simulink model "filtros_r2015b"  (R2015b)
settings: Solver=VariableStepAuto  SolverMode=SingleTasking  StartTime=0.0  StopTime=10.0  RelTol=1e-3
libraries: dsparch4 x4
(part 3 of 5)

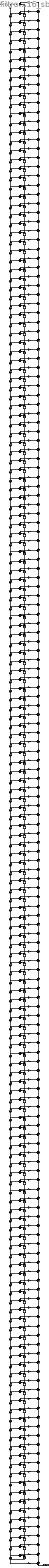
== system filtros_r2015b/filtro_bs_fir_direct_sym16_sb ==
  Input : Inport
  BodyDelayL{2..171} (170 alike) : Delay  DelayLength=1  InitialCondition=0
  BodyDelayR{2..171} (170 alike) : Delay  DelayLength=1  InitialCondition=0
  BodySumL{2..171} (170 alike) : Sum  Inputs=+|+  AccumDataTypeStr=fixdt(1,17,15)  OutDataTypeStr=fixdt(1,17,15)  RndMeth=Convergent
  BodySumR{2..171} (170 alike) : Sum  Inputs=++|  AccumDataTypeStr=fixdt(1,33,30)  OutDataTypeStr=fixdt(1,33,30)  RndMeth=Convergent
  ConvertIn : DataTypeConversion  OutDataTypeStr=fixdt(1,16,15)  RndMeth=Nearest  SaturateOnIntegerOverflow=on
  ConvertOut : DataTypeConversion  OutDataTypeStr=fixdt(1,33,30)  RndMeth=Convergent
  FootDelayL172 : Delay  DelayLength=1  InitialCondition=0
  FootSumR172 : Sum  Inputs=++|  AccumDataTypeStr=fixdt(1,33,30)  OutDataTypeStr=fixdt(1,33,30)  RndMeth=Convergent
  HeadDelayR1 : Delay  DelayLength=1  InitialCondition=0
  HeadSumL1 : Sum  Inputs=+|+  AccumDataTypeStr=fixdt(1,17,15)  OutDataTypeStr=fixdt(1,17,15)  RndMeth=Convergent
  h(1) : Gain  Gain=0.00222060902607300326  ParamDataTypeStr=fixdt(1,16,15)  OutDataTypeStr=fixdt(1,32,30)  RndMeth=Convergent
  h(10) : Gain  Gain=0.000412385856381775474  ParamDataTypeStr=fixdt(1,16,15)  OutDataTypeStr=fixdt(1,32,30)  RndMeth=Convergent
  h(100) : Gain  Gain=-0.00183683800817078082  ParamDataTypeStr=fixdt(1,16,15)  OutDataTypeStr=fixdt(1,32,30)  RndMeth=Convergent
  h(101) : Gain  Gain=-0.0108639596326587443  ParamDataTypeStr=fixdt(1,16,15)  OutDataTypeStr=fixdt(1,32,30)  RndMeth=Convergent
  h(102) : Gain  Gain=-0.00922719514825467643  ParamDataTypeStr=fixdt(1,16,15)  OutDataTypeStr=fixdt(1,32,30)  RndMeth=Convergent
  h(103) : Gain  Gain=0.00163747281524985618  ParamDataTypeStr=fixdt(1,16,15)  OutDataTypeStr=fixdt(1,32,30)  RndMeth=Convergent
  h(104) : Gain  Gain=0.0109887273848280828  ParamDataTypeStr=fixdt(1,16,15)  OutDataTypeStr=fixdt(1,32,30)  RndMeth=Convergent
  h(105) : Gain  Gain=0.00948674518474205107  ParamDataTypeStr=fixdt(1,16,15)  OutDataTypeStr=fixdt(1,32,30)  RndMeth=Convergent
  h(106) : Gain  Gain=-0.00138066436274078834  ParamDataTypeStr=fixdt(1,16,15)  OutDataTypeStr=fixdt(1,32,30)  RndMeth=Convergent
  h(107) : Gain  Gain=-0.0107847839373187305  ParamDataTypeStr=fixdt(1,16,15)  OutDataTypeStr=fixdt(1,32,30)  RndMeth=Convergent
  h(108) : Gain  Gain=-0.00943180866487196637  ParamDataTypeStr=fixdt(1,16,15)  OutDataTypeStr=fixdt(1,32,30)  RndMeth=Convergent
  h(109) : Gain  Gain=0.00112945650559354298  ParamDataTypeStr=fixdt(1,16,15)  OutDataTypeStr=fixdt(1,32,30)  RndMeth=Convergent
  h(11) : Gain  Gain=0.0012082136770825056  ParamDataTypeStr=fixdt(1,16,15)  OutDataTypeStr=fixdt(1,32,30)  RndMeth=Convergent
  h(110) : Gain  Gain=0.0102552016813565686  ParamDataTypeStr=fixdt(1,16,15)  OutDataTypeStr=fixdt(1,32,30)  RndMeth=Convergent
  h(111) : Gain  Gain=0.00900188398408828007  ParamDataTypeStr=fixdt(1,16,15)  OutDataTypeStr=fixdt(1,32,30)  RndMeth=Convergent
  h(112) : Gain  Gain=-0.000961145771569491512  ParamDataTypeStr=fixdt(1,16,15)  OutDataTypeStr=fixdt(1,32,30)  RndMeth=Convergent
  h(113) : Gain  Gain=-0.00942017850361522718  ParamDataTypeStr=fixdt(1,16,15)  OutDataTypeStr=fixdt(1,32,30)  RndMeth=Convergent
  h(114) : Gain  Gain=-0.00815339374212936327  ParamDataTypeStr=fixdt(1,16,15)  OutDataTypeStr=fixdt(1,32,30)  RndMeth=Convergent
  h(115) : Gain  Gain=0.00095452405654360248  ParamDataTypeStr=fixdt(1,16,15)  OutDataTypeStr=fixdt(1,32,30)  RndMeth=Convergent
  h(116) : Gain  Gain=0.00833604871664309077  ParamDataTypeStr=fixdt(1,16,15)  OutDataTypeStr=fixdt(1,32,30)  RndMeth=Convergent
  h(117) : Gain  Gain=0.00684396989036963662  ParamDataTypeStr=fixdt(1,16,15)  OutDataTypeStr=fixdt(1,32,30)  RndMeth=Convergent
  h(118) : Gain  Gain=-0.00119242778209114773  ParamDataTypeStr=fixdt(1,16,15)  OutDataTypeStr=fixdt(1,32,30)  RndMeth=Convergent
  h(119) : Gain  Gain=-0.00705305906451382351  ParamDataTypeStr=fixdt(1,16,15)  OutDataTypeStr=fixdt(1,32,30)  RndMeth=Convergent
  h(12) : Gain  Gain=0.000708848931376692445  ParamDataTypeStr=fixdt(1,16,15)  OutDataTypeStr=fixdt(1,32,30)  RndMeth=Convergent
  h(120) : Gain  Gain=-0.00507403810665585982  ParamDataTypeStr=fixdt(1,16,15)  OutDataTypeStr=fixdt(1,32,30)  RndMeth=Convergent
  h(121) : Gain  Gain=0.0017485040122219755  ParamDataTypeStr=fixdt(1,16,15)  OutDataTypeStr=fixdt(1,32,30)  RndMeth=Convergent
  h(122) : Gain  Gain=0.00566182762167975924  ParamDataTypeStr=fixdt(1,16,15)  OutDataTypeStr=fixdt(1,32,30)  RndMeth=Convergent
  h(123) : Gain  Gain=0.00285652374535125047  ParamDataTypeStr=fixdt(1,16,15)  OutDataTypeStr=fixdt(1,32,30)  RndMeth=Convergent
  h(124) : Gain  Gain=-0.00269106070621181808  ParamDataTypeStr=fixdt(1,16,15)  OutDataTypeStr=fixdt(1,32,30)  RndMeth=Convergent
  h(125) : Gain  Gain=-0.00424817527831348931  ParamDataTypeStr=fixdt(1,16,15)  OutDataTypeStr=fixdt(1,32,30)  RndMeth=Convergent
  h(126) : Gain  Gain=-0.000229684832746667594  ParamDataTypeStr=fixdt(1,16,15)  OutDataTypeStr=fixdt(1,32,30)  RndMeth=Convergent
  h(127) : Gain  Gain=0.00407093661353082233  ParamDataTypeStr=fixdt(1,16,15)  OutDataTypeStr=fixdt(1,32,30)  RndMeth=Convergent
  h(128) : Gain  Gain=0.00291483498180524067  ParamDataTypeStr=fixdt(1,16,15)  OutDataTypeStr=fixdt(1,32,30)  RndMeth=Convergent
  h(129) : Gain  Gain=-0.00274240933992378781  ParamDataTypeStr=fixdt(1,16,15)  OutDataTypeStr=fixdt(1,32,30)  RndMeth=Convergent
  h(13) : Gain  Gain=-0.000527267715872998242  ParamDataTypeStr=fixdt(1,16,15)  OutDataTypeStr=fixdt(1,32,30)  RndMeth=Convergent
  h(130) : Gain  Gain=-0.00591588442091149896  ParamDataTypeStr=fixdt(1,16,15)  OutDataTypeStr=fixdt(1,32,30)  RndMeth=Convergent
  h(131) : Gain  Gain=-0.0017616838703545161  ParamDataTypeStr=fixdt(1,16,15)  OutDataTypeStr=fixdt(1,32,30)  RndMeth=Convergent
  h(132) : Gain  Gain=0.00597490325309535299  ParamDataTypeStr=fixdt(1,16,15)  OutDataTypeStr=fixdt(1,32,30)  RndMeth=Convergent
  h(133) : Gain  Gain=0.00823416750476205564  ParamDataTypeStr=fixdt(1,16,15)  OutDataTypeStr=fixdt(1,32,30)  RndMeth=Convergent
  h(134) : Gain  Gain=0.000885427072030269056  ParamDataTypeStr=fixdt(1,16,15)  OutDataTypeStr=fixdt(1,32,30)  RndMeth=Convergent
  h(135) : Gain  Gain=-0.0093650338513660801  ParamDataTypeStr=fixdt(1,16,15)  OutDataTypeStr=fixdt(1,32,30)  RndMeth=Convergent
  h(136) : Gain  Gain=-0.0110087803321226481  ParamDataTypeStr=fixdt(1,16,15)  OutDataTypeStr=fixdt(1,32,30)  RndMeth=Convergent
  h(137) : Gain  Gain=-0.000374405366293637204  ParamDataTypeStr=fixdt(1,16,15)  OutDataTypeStr=fixdt(1,32,30)  RndMeth=Convergent
  h(138) : Gain  Gain=0.0127923118217058915  ParamDataTypeStr=fixdt(1,16,15)  OutDataTypeStr=fixdt(1,32,30)  RndMeth=Convergent
  h(139) : Gain  Gain=0.0141925500900669105  ParamDataTypeStr=fixdt(1,16,15)  OutDataTypeStr=fixdt(1,32,30)  RndMeth=Convergent
  h(14) : Gain  Gain=-0.00115435994390551471  ParamDataTypeStr=fixdt(1,16,15)  OutDataTypeStr=fixdt(1,32,30)  RndMeth=Convergent
  h(140) : Gain  Gain=0.000297609131461152134  ParamDataTypeStr=fixdt(1,16,15)  OutDataTypeStr=fixdt(1,32,30)  RndMeth=Convergent
  h(141) : Gain  Gain=-0.0161298900491302633  ParamDataTypeStr=fixdt(1,16,15)  OutDataTypeStr=fixdt(1,32,30)  RndMeth=Convergent
  h(142) : Gain  Gain=-0.0177117572182131991  ParamDataTypeStr=fixdt(1,16,15)  OutDataTypeStr=fixdt(1,32,30)  RndMeth=Convergent
  h(143) : Gain  Gain=-0.00070122210733707406  ParamDataTypeStr=fixdt(1,16,15)  OutDataTypeStr=fixdt(1,32,30)  RndMeth=Convergent
  h(144) : Gain  Gain=0.0192516530564409392  ParamDataTypeStr=fixdt(1,16,15)  OutDataTypeStr=fixdt(1,32,30)  RndMeth=Convergent
  h(145) : Gain  Gain=0.0214725815198791338  ParamDataTypeStr=fixdt(1,16,15)  OutDataTypeStr=fixdt(1,32,30)  RndMeth=Convergent
  h(146) : Gain  Gain=0.00160886427991767172  ParamDataTypeStr=fixdt(1,16,15)  OutDataTypeStr=fixdt(1,32,30)  RndMeth=Convergent
  h(147) : Gain  Gain=-0.0220352330154781964  ParamDataTypeStr=fixdt(1,16,15)  OutDataTypeStr=fixdt(1,32,30)  RndMeth=Convergent
  h(148) : Gain  Gain=-0.0253625767260405761  ParamDataTypeStr=fixdt(1,16,15)  OutDataTypeStr=fixdt(1,32,30)  RndMeth=Convergent
  h(149) : Gain  Gain=-0.00302084071867347913  ParamDataTypeStr=fixdt(1,16,15)  OutDataTypeStr=fixdt(1,32,30)  RndMeth=Convergent
  h(15) : Gain  Gain=-0.000500072760209519418  ParamDataTypeStr=fixdt(1,16,15)  OutDataTypeStr=fixdt(1,32,30)  RndMeth=Convergent
  h(150) : Gain  Gain=0.0243632351958552353  ParamDataTypeStr=fixdt(1,16,15)  OutDataTypeStr=fixdt(1,32,30)  RndMeth=Convergent
  h(151) : Gain  Gain=0.0292458735180988298  ParamDataTypeStr=fixdt(1,16,15)  OutDataTypeStr=fixdt(1,32,30)  RndMeth=Convergent
  h(152) : Gain  Gain=0.00489806445322205682  ParamDataTypeStr=fixdt(1,16,15)  OutDataTypeStr=fixdt(1,32,30)  RndMeth=Convergent
  h(153) : Gain  Gain=-0.0261477012653955863  ParamDataTypeStr=fixdt(1,16,15)  OutDataTypeStr=fixdt(1,32,30)  RndMeth=Convergent
  h(154) : Gain  Gain=-0.0329897200285691264  ParamDataTypeStr=fixdt(1,16,15)  OutDataTypeStr=fixdt(1,32,30)  RndMeth=Convergent
  h(155) : Gain  Gain=-0.00718491130158882118  ParamDataTypeStr=fixdt(1,16,15)  OutDataTypeStr=fixdt(1,32,30)  RndMeth=Convergent
  h(156) : Gain  Gain=0.0273141193534726101  ParamDataTypeStr=fixdt(1,16,15)  OutDataTypeStr=fixdt(1,32,30)  RndMeth=Convergent
  h(157) : Gain  Gain=0.0364508104956247289  ParamDataTypeStr=fixdt(1,16,15)  OutDataTypeStr=fixdt(1,32,30)  RndMeth=Convergent
  h(158) : Gain  Gain=0.00979190705266517157  ParamDataTypeStr=fixdt(1,16,15)  OutDataTypeStr=fixdt(1,32,30)  RndMeth=Convergent
  h(159) : Gain  Gain=-0.0278216938080646271  ParamDataTypeStr=fixdt(1,16,15)  OutDataTypeStr=fixdt(1,32,30)  RndMeth=Convergent
  h(16) : Gain  Gain=0.000688761844683712598  ParamDataTypeStr=fixdt(1,16,15)  OutDataTypeStr=fixdt(1,32,30)  RndMeth=Convergent
  h(160) : Gain  Gain=-0.0394970137823456025  ParamDataTypeStr=fixdt(1,16,15)  OutDataTypeStr=fixdt(1,32,30)  RndMeth=Convergent
  h(161) : Gain  Gain=-0.0126125709016341354  ParamDataTypeStr=fixdt(1,16,15)  OutDataTypeStr=fixdt(1,32,30)  RndMeth=Convergent
  h(162) : Gain  Gain=0.0276570288609940609  ParamDataTypeStr=fixdt(1,16,15)  OutDataTypeStr=fixdt(1,32,30)  RndMeth=Convergent
  h(163) : Gain  Gain=0.0420062041083570439  ParamDataTypeStr=fixdt(1,16,15)  OutDataTypeStr=fixdt(1,32,30)  RndMeth=Convergent
  h(164) : Gain  Gain=0.0155224470683002526  ParamDataTypeStr=fixdt(1,16,15)  OutDataTypeStr=fixdt(1,32,30)  RndMeth=Convergent
  h(165) : Gain  Gain=-0.0268379125320710073  ParamDataTypeStr=fixdt(1,16,15)  OutDataTypeStr=fixdt(1,32,30)  RndMeth=Convergent
  h(166) : Gain  Gain=-0.0438767987017301478  ParamDataTypeStr=fixdt(1,16,15)  OutDataTypeStr=fixdt(1,32,30)  RndMeth=Convergent
  h(167) : Gain  Gain=-0.0183901617907575449  ParamDataTypeStr=fixdt(1,16,15)  OutDataTypeStr=fixdt(1,32,30)  RndMeth=Convergent
  h(168) : Gain  Gain=0.0254141122423833764  ParamDataTypeStr=fixdt(1,16,15)  OutDataTypeStr=fixdt(1,32,30)  RndMeth=Convergent
  h(169) : Gain  Gain=0.0450290877668963474  ParamDataTypeStr=fixdt(1,16,15)  OutDataTypeStr=fixdt(1,32,30)  RndMeth=Convergent
  h(17) : Gain  Gain=0.00107522738688104608  ParamDataTypeStr=fixdt(1,16,15)  OutDataTypeStr=fixdt(1,32,30)  RndMeth=Convergent
  h(170) : Gain  Gain=0.021081893690384497  ParamDataTypeStr=fixdt(1,16,15)  OutDataTypeStr=fixdt(1,32,30)  RndMeth=Convergent
  h(171) : Gain  Gain=-0.0234612272015558634  ParamDataTypeStr=fixdt(1,16,15)  OutDataTypeStr=fixdt(1,32,30)  RndMeth=Convergent
  h(172) : Gain  Gain=0.92844636087036847  ParamDataTypeStr=fixdt(1,16,15)  OutDataTypeStr=fixdt(1,32,30)  RndMeth=Convergent
  h(18) : Gain  Gain=0.00021708622303679784  ParamDataTypeStr=fixdt(1,16,15)  OutDataTypeStr=fixdt(1,32,30)  RndMeth=Convergent
  h(19) : Gain  Gain=-0.000907506893595811152  ParamDataTypeStr=fixdt(1,16,15)  OutDataTypeStr=fixdt(1,32,30)  RndMeth=Convergent
  h(2) : Gain  Gain=-0.0126542523812769661  ParamDataTypeStr=fixdt(1,16,15)  OutDataTypeStr=fixdt(1,32,30)  RndMeth=Convergent
  h(20) : Gain  Gain=-0.00098456841772494026  ParamDataTypeStr=fixdt(1,16,15)  OutDataTypeStr=fixdt(1,32,30)  RndMeth=Convergent
  h(21) : Gain  Gain=0.000135034611801735488  ParamDataTypeStr=fixdt(1,16,15)  OutDataTypeStr=fixdt(1,32,30)  RndMeth=Convergent
  h(22) : Gain  Gain=0.0011904117302944002  ParamDataTypeStr=fixdt(1,16,15)  OutDataTypeStr=fixdt(1,32,30)  RndMeth=Convergent
  h(23) : Gain  Gain=0.000897348105847610368  ParamDataTypeStr=fixdt(1,16,15)  OutDataTypeStr=fixdt(1,32,30)  RndMeth=Convergent
  h(24) : Gain  Gain=-0.000544809004851308965  ParamDataTypeStr=fixdt(1,16,15)  OutDataTypeStr=fixdt(1,32,30)  RndMeth=Convergent
  h(25) : Gain  Gain=-0.00153935391414636888  ParamDataTypeStr=fixdt(1,16,15)  OutDataTypeStr=fixdt(1,32,30)  RndMeth=Convergent
  h(26) : Gain  Gain=-0.000828005173735774504  ParamDataTypeStr=fixdt(1,16,15)  OutDataTypeStr=fixdt(1,32,30)  RndMeth=Convergent
  h(27) : Gain  Gain=0.000996889815879576074  ParamDataTypeStr=fixdt(1,16,15)  OutDataTypeStr=fixdt(1,32,30)  RndMeth=Convergent
  h(28) : Gain  Gain=0.0019514135346378515  ParamDataTypeStr=fixdt(1,16,15)  OutDataTypeStr=fixdt(1,32,30)  RndMeth=Convergent
  h(29) : Gain  Gain=0.000790406883380305979  ParamDataTypeStr=fixdt(1,16,15)  OutDataTypeStr=fixdt(1,32,30)  RndMeth=Convergent
  h(3) : Gain  Gain=-0.00285785975806639734  ParamDataTypeStr=fixdt(1,16,15)  OutDataTypeStr=fixdt(1,32,30)  RndMeth=Convergent
  h(30) : Gain  Gain=-0.00147057635761781201  ParamDataTypeStr=fixdt(1,16,15)  OutDataTypeStr=fixdt(1,32,30)  RndMeth=Convergent
  h(31) : Gain  Gain=-0.00241626228825247806  ParamDataTypeStr=fixdt(1,16,15)  OutDataTypeStr=fixdt(1,32,30)  RndMeth=Convergent
  h(32) : Gain  Gain=-0.00079322658642497451  ParamDataTypeStr=fixdt(1,16,15)  OutDataTypeStr=fixdt(1,32,30)  RndMeth=Convergent
  h(33) : Gain  Gain=0.00194526333770608968  ParamDataTypeStr=fixdt(1,16,15)  OutDataTypeStr=fixdt(1,32,30)  RndMeth=Convergent
  h(34) : Gain  Gain=0.0029194310934874913  ParamDataTypeStr=fixdt(1,16,15)  OutDataTypeStr=fixdt(1,32,30)  RndMeth=Convergent
  h(35) : Gain  Gain=0.000842470514714747172  ParamDataTypeStr=fixdt(1,16,15)  OutDataTypeStr=fixdt(1,32,30)  RndMeth=Convergent
  h(36) : Gain  Gain=-0.00239778430088512153  ParamDataTypeStr=fixdt(1,16,15)  OutDataTypeStr=fixdt(1,32,30)  RndMeth=Convergent
  h(37) : Gain  Gain=-0.00343927344050146957  ParamDataTypeStr=fixdt(1,16,15)  OutDataTypeStr=fixdt(1,32,30)  RndMeth=Convergent
  h(38) : Gain  Gain=-0.000936473940016707435  ParamDataTypeStr=fixdt(1,16,15)  OutDataTypeStr=fixdt(1,32,30)  RndMeth=Convergent
  h(39) : Gain  Gain=0.00280722916414461419  ParamDataTypeStr=fixdt(1,16,15)  OutDataTypeStr=fixdt(1,32,30)  RndMeth=Convergent
  h(4) : Gain  Gain=-6.27866860752195359e-05  ParamDataTypeStr=fixdt(1,16,15)  OutDataTypeStr=fixdt(1,32,30)  RndMeth=Convergent
  h(40) : Gain  Gain=0.00395010111825385129  ParamDataTypeStr=fixdt(1,16,15)  OutDataTypeStr=fixdt(1,32,30)  RndMeth=Convergent
  h(41) : Gain  Gain=0.00106808840411088692  ParamDataTypeStr=fixdt(1,16,15)  OutDataTypeStr=fixdt(1,32,30)  RndMeth=Convergent
  h(42) : Gain  Gain=-0.00315451566029618024  ParamDataTypeStr=fixdt(1,16,15)  OutDataTypeStr=fixdt(1,32,30)  RndMeth=Convergent
  h(43) : Gain  Gain=-0.00442195264195982887  ParamDataTypeStr=fixdt(1,16,15)  OutDataTypeStr=fixdt(1,32,30)  RndMeth=Convergent
  h(44) : Gain  Gain=-0.00122255919972922753  ParamDataTypeStr=fixdt(1,16,15)  OutDataTypeStr=fixdt(1,32,30)  RndMeth=Convergent
  h(45) : Gain  Gain=0.00342517772747777133  ParamDataTypeStr=fixdt(1,16,15)  OutDataTypeStr=fixdt(1,32,30)  RndMeth=Convergent
  h(46) : Gain  Gain=0.00482320302455260287  ParamDataTypeStr=fixdt(1,16,15)  OutDataTypeStr=fixdt(1,32,30)  RndMeth=Convergent
  h(47) : Gain  Gain=0.00137963206631302971  ParamDataTypeStr=fixdt(1,16,15)  OutDataTypeStr=fixdt(1,32,30)  RndMeth=Convergent
  h(48) : Gain  Gain=-0.00361108914948540588  ParamDataTypeStr=fixdt(1,16,15)  OutDataTypeStr=fixdt(1,32,30)  RndMeth=Convergent
  h(49) : Gain  Gain=-0.0051234196132662101  ParamDataTypeStr=fixdt(1,16,15)  OutDataTypeStr=fixdt(1,32,30)  RndMeth=Convergent
  h(5) : Gain  Gain=0.0011441808540458725  ParamDataTypeStr=fixdt(1,16,15)  OutDataTypeStr=fixdt(1,32,30)  RndMeth=Convergent
  h(50) : Gain  Gain=-0.00151391720299139305  ParamDataTypeStr=fixdt(1,16,15)  OutDataTypeStr=fixdt(1,32,30)  RndMeth=Convergent
  h(51) : Gain  Gain=0.00370986731030357791  ParamDataTypeStr=fixdt(1,16,15)  OutDataTypeStr=fixdt(1,32,30)  RndMeth=Convergent
  h(52) : Gain  Gain=0.00529509616594016613  ParamDataTypeStr=fixdt(1,16,15)  OutDataTypeStr=fixdt(1,32,30)  RndMeth=Convergent
  h(53) : Gain  Gain=0.00159648812698948606  ParamDataTypeStr=fixdt(1,16,15)  OutDataTypeStr=fixdt(1,32,30)  RndMeth=Convergent
  h(54) : Gain  Gain=-0.00373099483536572154  ParamDataTypeStr=fixdt(1,16,15)  OutDataTypeStr=fixdt(1,32,30)  RndMeth=Convergent
  h(55) : Gain  Gain=-0.00532117775878846073  ParamDataTypeStr=fixdt(1,16,15)  OutDataTypeStr=fixdt(1,32,30)  RndMeth=Convergent
  h(56) : Gain  Gain=-0.00159242660687583873  ParamDataTypeStr=fixdt(1,16,15)  OutDataTypeStr=fixdt(1,32,30)  RndMeth=Convergent
  h(57) : Gain  Gain=0.00367945523701494748  ParamDataTypeStr=fixdt(1,16,15)  OutDataTypeStr=fixdt(1,32,30)  RndMeth=Convergent
  h(58) : Gain  Gain=0.0052061653709269606  ParamDataTypeStr=fixdt(1,16,15)  OutDataTypeStr=fixdt(1,32,30)  RndMeth=Convergent
  h(59) : Gain  Gain=0.00147157392126652845  ParamDataTypeStr=fixdt(1,16,15)  OutDataTypeStr=fixdt(1,32,30)  RndMeth=Convergent
  h(6) : Gain  Gain=0.000896258283817716328  ParamDataTypeStr=fixdt(1,16,15)  OutDataTypeStr=fixdt(1,32,30)  RndMeth=Convergent
  h(60) : Gain  Gain=-0.00361588185118073922  ParamDataTypeStr=fixdt(1,16,15)  OutDataTypeStr=fixdt(1,32,30)  RndMeth=Convergent
  h(61) : Gain  Gain=-0.00490141555871920903  ParamDataTypeStr=fixdt(1,16,15)  OutDataTypeStr=fixdt(1,32,30)  RndMeth=Convergent
  h(62) : Gain  Gain=-0.00121047830165690374  ParamDataTypeStr=fixdt(1,16,15)  OutDataTypeStr=fixdt(1,32,30)  RndMeth=Convergent
  h(63) : Gain  Gain=0.00352542594050439051  ParamDataTypeStr=fixdt(1,16,15)  OutDataTypeStr=fixdt(1,32,30)  RndMeth=Convergent
  h(64) : Gain  Gain=0.00445284916134371014  ParamDataTypeStr=fixdt(1,16,15)  OutDataTypeStr=fixdt(1,32,30)  RndMeth=Convergent
  h(65) : Gain  Gain=0.000791426268911049158  ParamDataTypeStr=fixdt(1,16,15)  OutDataTypeStr=fixdt(1,32,30)  RndMeth=Convergent
  h(66) : Gain  Gain=-0.00345955811828613236  ParamDataTypeStr=fixdt(1,16,15)  OutDataTypeStr=fixdt(1,32,30)  RndMeth=Convergent
  h(67) : Gain  Gain=-0.00386295620000698219  ParamDataTypeStr=fixdt(1,16,15)  OutDataTypeStr=fixdt(1,32,30)  RndMeth=Convergent
  h(68) : Gain  Gain=-0.000195973685172349036  ParamDataTypeStr=fixdt(1,16,15)  OutDataTypeStr=fixdt(1,32,30)  RndMeth=Convergent
  h(69) : Gain  Gain=0.00344274784340699606  ParamDataTypeStr=fixdt(1,16,15)  OutDataTypeStr=fixdt(1,32,30)  RndMeth=Convergent
  h(7) : Gain  Gain=-0.000331426495396970144  ParamDataTypeStr=fixdt(1,16,15)  OutDataTypeStr=fixdt(1,32,30)  RndMeth=Convergent
  h(70) : Gain  Gain=0.00315382863405564307  ParamDataTypeStr=fixdt(1,16,15)  OutDataTypeStr=fixdt(1,32,30)  RndMeth=Convergent
  h(71) : Gain  Gain=-0.000582376133074710006  ParamDataTypeStr=fixdt(1,16,15)  OutDataTypeStr=fixdt(1,32,30)  RndMeth=Convergent
  h(72) : Gain  Gain=-0.00351181599169146652  ParamDataTypeStr=fixdt(1,16,15)  OutDataTypeStr=fixdt(1,32,30)  RndMeth=Convergent
  h(73) : Gain  Gain=-0.00236215784465629297  ParamDataTypeStr=fixdt(1,16,15)  OutDataTypeStr=fixdt(1,32,30)  RndMeth=Convergent
  h(74) : Gain  Gain=0.00153579939763267333  ParamDataTypeStr=fixdt(1,16,15)  OutDataTypeStr=fixdt(1,32,30)  RndMeth=Convergent
  h(75) : Gain  Gain=0.00370136458943965373  ParamDataTypeStr=fixdt(1,16,15)  OutDataTypeStr=fixdt(1,32,30)  RndMeth=Convergent
  h(76) : Gain  Gain=0.00154425151614053543  ParamDataTypeStr=fixdt(1,16,15)  OutDataTypeStr=fixdt(1,32,30)  RndMeth=Convergent
  h(77) : Gain  Gain=-0.00262336900807332929  ParamDataTypeStr=fixdt(1,16,15)  OutDataTypeStr=fixdt(1,32,30)  RndMeth=Convergent
  h(78) : Gain  Gain=-0.00400604629593016501  ParamDataTypeStr=fixdt(1,16,15)  OutDataTypeStr=fixdt(1,32,30)  RndMeth=Convergent
  h(79) : Gain  Gain=-0.000720258293274521409  ParamDataTypeStr=fixdt(1,16,15)  OutDataTypeStr=fixdt(1,32,30)  RndMeth=Convergent
  h(8) : Gain  Gain=-0.00122625529434006045  ParamDataTypeStr=fixdt(1,16,15)  OutDataTypeStr=fixdt(1,32,30)  RndMeth=Convergent
  h(80) : Gain  Gain=0.00383463380064707733  ParamDataTypeStr=fixdt(1,16,15)  OutDataTypeStr=fixdt(1,32,30)  RndMeth=Convergent
  h(81) : Gain  Gain=0.00445475536974668761  ParamDataTypeStr=fixdt(1,16,15)  OutDataTypeStr=fixdt(1,32,30)  RndMeth=Convergent
  h(82) : Gain  Gain=-4.60177465353575697e-05  ParamDataTypeStr=fixdt(1,16,15)  OutDataTypeStr=fixdt(1,32,30)  RndMeth=Convergent
  h(83) : Gain  Gain=-0.00510941162252769206  ParamDataTypeStr=fixdt(1,16,15)  OutDataTypeStr=fixdt(1,32,30)  RndMeth=Convergent
  h(84) : Gain  Gain=-0.00503113887403160848  ParamDataTypeStr=fixdt(1,16,15)  OutDataTypeStr=fixdt(1,32,30)  RndMeth=Convergent
  h(85) : Gain  Gain=0.000719907321048572049  ParamDataTypeStr=fixdt(1,16,15)  OutDataTypeStr=fixdt(1,32,30)  RndMeth=Convergent
  h(86) : Gain  Gain=0.00639742929747593846  ParamDataTypeStr=fixdt(1,16,15)  OutDataTypeStr=fixdt(1,32,30)  RndMeth=Convergent
  h(87) : Gain  Gain=0.00571934912806121212  ParamDataTypeStr=fixdt(1,16,15)  OutDataTypeStr=fixdt(1,32,30)  RndMeth=Convergent
  h(88) : Gain  Gain=-0.00126357426321187542  ParamDataTypeStr=fixdt(1,16,15)  OutDataTypeStr=fixdt(1,32,30)  RndMeth=Convergent
  h(89) : Gain  Gain=-0.00763605641798632221  ParamDataTypeStr=fixdt(1,16,15)  OutDataTypeStr=fixdt(1,32,30)  RndMeth=Convergent
  h(9) : Gain  Gain=-0.000842143561281415501  ParamDataTypeStr=fixdt(1,16,15)  OutDataTypeStr=fixdt(1,32,30)  RndMeth=Convergent
  h(90) : Gain  Gain=-0.00648525362000833966  ParamDataTypeStr=fixdt(1,16,15)  OutDataTypeStr=fixdt(1,32,30)  RndMeth=Convergent
  h(91) : Gain  Gain=0.00165155190893082971  ParamDataTypeStr=fixdt(1,16,15)  OutDataTypeStr=fixdt(1,32,30)  RndMeth=Convergent
  h(92) : Gain  Gain=0.00876118917065600751  ParamDataTypeStr=fixdt(1,16,15)  OutDataTypeStr=fixdt(1,32,30)  RndMeth=Convergent
  h(93) : Gain  Gain=0.0072820300968526562  ParamDataTypeStr=fixdt(1,16,15)  OutDataTypeStr=fixdt(1,32,30)  RndMeth=Convergent
  h(94) : Gain  Gain=-0.00187150944773054636  ParamDataTypeStr=fixdt(1,16,15)  OutDataTypeStr=fixdt(1,32,30)  RndMeth=Convergent
  h(95) : Gain  Gain=-0.00971025998510001952  ParamDataTypeStr=fixdt(1,16,15)  OutDataTypeStr=fixdt(1,32,30)  RndMeth=Convergent
  h(96) : Gain  Gain=-0.00805071853330361492  ParamDataTypeStr=fixdt(1,16,15)  OutDataTypeStr=fixdt(1,32,30)  RndMeth=Convergent
  h(97) : Gain  Gain=0.00192657035016093937  ParamDataTypeStr=fixdt(1,16,15)  OutDataTypeStr=fixdt(1,32,30)  RndMeth=Convergent
  h(98) : Gain  Gain=0.0104266340022652303  ParamDataTypeStr=fixdt(1,16,15)  OutDataTypeStr=fixdt(1,32,30)  RndMeth=Convergent
  h(99) : Gain  Gain=0.00872346674455828572  ParamDataTypeStr=fixdt(1,16,15)  OutDataTypeStr=fixdt(1,32,30)  RndMeth=Convergent
  Output : Outport
  wires:
  Input/1 -> ConvertIn/1
  HeadSumL1/1 -> h(1)/1
  h(1)/1 -> BodySumR2/2
  HeadDelayR1/1 -> HeadSumL1/2
  ConvertIn/1 -> HeadSumL1/1, BodyDelayL2/1
  BodyDelayL2/1 -> BodySumL2/1, BodyDelayL3/1
  BodySumL2/1 -> h(2)/1
  h(2)/1 -> BodySumR2/1
  BodyDelayR2/1 -> BodySumL2/2, HeadDelayR1/1
  BodySumR2/1 -> BodySumR3/2
  BodyDelayL3/1 -> BodySumL3/1, BodyDelayL4/1
  BodySumL3/1 -> h(3)/1
  h(3)/1 -> BodySumR3/1
  BodyDelayR3/1 -> BodySumL3/2, BodyDelayR2/1
  BodySumR3/1 -> BodySumR4/2
  BodyDelayL4/1 -> BodySumL4/1, BodyDelayL5/1
  BodySumL4/1 -> h(4)/1
  h(4)/1 -> BodySumR4/1
  BodyDelayR4/1 -> BodySumL4/2, BodyDelayR3/1
  BodySumR4/1 -> BodySumR5/2
  BodyDelayL5/1 -> BodySumL5/1, BodyDelayL6/1
  BodySumL5/1 -> h(5)/1
  h(5)/1 -> BodySumR5/1
  BodyDelayR5/1 -> BodySumL5/2, BodyDelayR4/1
  BodySumR5/1 -> BodySumR6/2
  BodyDelayL6/1 -> BodySumL6/1, BodyDelayL7/1
  BodySumL6/1 -> h(6)/1
  h(6)/1 -> BodySumR6/1
  BodyDelayR6/1 -> BodySumL6/2, BodyDelayR5/1
  BodySumR6/1 -> BodySumR7/2
  BodyDelayL7/1 -> BodySumL7/1, BodyDelayL8/1
  BodySumL7/1 -> h(7)/1
  h(7)/1 -> BodySumR7/1
  BodyDelayR7/1 -> BodySumL7/2, BodyDelayR6/1
  BodySumR7/1 -> BodySumR8/2
  BodyDelayL8/1 -> BodySumL8/1, BodyDelayL9/1
  BodySumL8/1 -> h(8)/1
  h(8)/1 -> BodySumR8/1
  BodyDelayR8/1 -> BodySumL8/2, BodyDelayR7/1
  BodySumR8/1 -> BodySumR9/2
  BodyDelayL9/1 -> BodySumL9/1, BodyDelayL10/1
  BodySumL9/1 -> h(9)/1
  h(9)/1 -> BodySumR9/1
  BodyDelayR9/1 -> BodySumL9/2, BodyDelayR8/1
  BodySumR9/1 -> BodySumR10/2
  BodyDelayL10/1 -> BodySumL10/1, BodyDelayL11/1
  BodySumL10/1 -> h(10)/1
  h(10)/1 -> BodySumR10/1
  BodyDelayR10/1 -> BodySumL10/2, BodyDelayR9/1
  BodySumR10/1 -> BodySumR11/2
  BodyDelayL11/1 -> BodySumL11/1, BodyDelayL12/1
  BodySumL11/1 -> h(11)/1
  h(11)/1 -> BodySumR11/1
  BodyDelayR11/1 -> BodySumL11/2, BodyDelayR10/1
  BodySumR11/1 -> BodySumR12/2
  BodyDelayL12/1 -> BodySumL12/1, BodyDelayL13/1
  BodySumL12/1 -> h(12)/1
  h(12)/1 -> BodySumR12/1
  BodyDelayR12/1 -> BodySumL12/2, BodyDelayR11/1
  BodySumR12/1 -> BodySumR13/2
  BodyDelayL13/1 -> BodySumL13/1, BodyDelayL14/1
  BodySumL13/1 -> h(13)/1
  h(13)/1 -> BodySumR13/1
  BodyDelayR13/1 -> BodySumL13/2, BodyDelayR12/1
  BodySumR13/1 -> BodySumR14/2
  BodyDelayL14/1 -> BodySumL14/1, BodyDelayL15/1
  BodySumL14/1 -> h(14)/1
  h(14)/1 -> BodySumR14/1
  BodyDelayR14/1 -> BodySumL14/2, BodyDelayR13/1
  BodySumR14/1 -> BodySumR15/2
  BodyDelayL15/1 -> BodySumL15/1, BodyDelayL16/1
  BodySumL15/1 -> h(15)/1
  h(15)/1 -> BodySumR15/1
  BodyDelayR15/1 -> BodySumL15/2, BodyDelayR14/1
  BodySumR15/1 -> BodySumR16/2
  BodyDelayL16/1 -> BodySumL16/1, BodyDelayL17/1
  BodySumL16/1 -> h(16)/1
  h(16)/1 -> BodySumR16/1
  BodyDelayR16/1 -> BodySumL16/2, BodyDelayR15/1
  BodySumR16/1 -> BodySumR17/2
  BodyDelayL17/1 -> BodySumL17/1, BodyDelayL18/1
  BodySumL17/1 -> h(17)/1
  h(17)/1 -> BodySumR17/1
  BodyDelayR17/1 -> BodySumL17/2, BodyDelayR16/1
  BodySumR17/1 -> BodySumR18/2
  BodyDelayL18/1 -> BodySumL18/1, BodyDelayL19/1
  BodySumL18/1 -> h(18)/1
  h(18)/1 -> BodySumR18/1
  BodyDelayR18/1 -> BodySumL18/2, BodyDelayR17/1
  BodySumR18/1 -> BodySumR19/2
  BodyDelayL19/1 -> BodySumL19/1, BodyDelayL20/1
  BodySumL19/1 -> h(19)/1
  h(19)/1 -> BodySumR19/1
  BodyDelayR19/1 -> BodySumL19/2, BodyDelayR18/1
  BodySumR19/1 -> BodySumR20/2
  BodyDelayL20/1 -> BodySumL20/1, BodyDelayL21/1
  BodySumL20/1 -> h(20)/1
  h(20)/1 -> BodySumR20/1
  BodyDelayR20/1 -> BodySumL20/2, BodyDelayR19/1
  BodySumR20/1 -> BodySumR21/2
  BodyDelayL21/1 -> BodySumL21/1, BodyDelayL22/1
  BodySumL21/1 -> h(21)/1
  h(21)/1 -> BodySumR21/1
  BodyDelayR21/1 -> BodySumL21/2, BodyDelayR20/1
  BodySumR21/1 -> BodySumR22/2
  BodyDelayL22/1 -> BodySumL22/1, BodyDelayL23/1
  BodySumL22/1 -> h(22)/1
  h(22)/1 -> BodySumR22/1
  BodyDelayR22/1 -> BodySumL22/2, BodyDelayR21/1
  BodySumR22/1 -> BodySumR23/2
  BodyDelayL23/1 -> BodySumL23/1, BodyDelayL24/1
  BodySumL23/1 -> h(23)/1
  h(23)/1 -> BodySumR23/1
  BodyDelayR23/1 -> BodySumL23/2, BodyDelayR22/1
  BodySumR23/1 -> BodySumR24/2
  BodyDelayL24/1 -> BodySumL24/1, BodyDelayL25/1
  BodySumL24/1 -> h(24)/1
  h(24)/1 -> BodySumR24/1
  BodyDelayR24/1 -> BodySumL24/2, BodyDelayR23/1
  BodySumR24/1 -> BodySumR25/2
  BodyDelayL25/1 -> BodySumL25/1, BodyDelayL26/1
  BodySumL25/1 -> h(25)/1
  h(25)/1 -> BodySumR25/1
  BodyDelayR25/1 -> BodySumL25/2, BodyDelayR24/1
  BodySumR25/1 -> BodySumR26/2
  BodyDelayL26/1 -> BodySumL26/1, BodyDelayL27/1
  BodySumL26/1 -> h(26)/1
  h(26)/1 -> BodySumR26/1
  BodyDelayR26/1 -> BodySumL26/2, BodyDelayR25/1
  BodySumR26/1 -> BodySumR27/2
  BodyDelayL27/1 -> BodySumL27/1, BodyDelayL28/1
  BodySumL27/1 -> h(27)/1
  h(27)/1 -> BodySumR27/1
  BodyDelayR27/1 -> BodySumL27/2, BodyDelayR26/1
  BodySumR27/1 -> BodySumR28/2
  BodyDelayL28/1 -> BodySumL28/1, BodyDelayL29/1
  BodySumL28/1 -> h(28)/1
  h(28)/1 -> BodySumR28/1
  BodyDelayR28/1 -> BodySumL28/2, BodyDelayR27/1
  BodySumR28/1 -> BodySumR29/2
  BodyDelayL29/1 -> BodySumL29/1, BodyDelayL30/1
  BodySumL29/1 -> h(29)/1
  h(29)/1 -> BodySumR29/1
  BodyDelayR29/1 -> BodySumL29/2, BodyDelayR28/1
  BodySumR29/1 -> BodySumR30/2
  BodyDelayL30/1 -> BodySumL30/1, BodyDelayL31/1
  BodySumL30/1 -> h(30)/1
  h(30)/1 -> BodySumR30/1
  BodyDelayR30/1 -> BodySumL30/2, BodyDelayR29/1
  BodySumR30/1 -> BodySumR31/2
  BodyDelayL31/1 -> BodySumL31/1, BodyDelayL32/1
  BodySumL31/1 -> h(31)/1
  h(31)/1 -> BodySumR31/1
  BodyDelayR31/1 -> BodySumL31/2, BodyDelayR30/1
  BodySumR31/1 -> BodySumR32/2
  BodyDelayL32/1 -> BodySumL32/1, BodyDelayL33/1
  BodySumL32/1 -> h(32)/1
  h(32)/1 -> BodySumR32/1
  BodyDelayR32/1 -> BodySumL32/2, BodyDelayR31/1
  BodySumR32/1 -> BodySumR33/2
  BodyDelayL33/1 -> BodySumL33/1, BodyDelayL34/1
  BodySumL33/1 -> h(33)/1
  h(33)/1 -> BodySumR33/1
  BodyDelayR33/1 -> BodySumL33/2, BodyDelayR32/1
  BodySumR33/1 -> BodySumR34/2
  BodyDelayL34/1 -> BodySumL34/1, BodyDelayL35/1
  BodySumL34/1 -> h(34)/1
  h(34)/1 -> BodySumR34/1
  BodyDelayR34/1 -> BodySumL34/2, BodyDelayR33/1
  BodySumR34/1 -> BodySumR35/2
  BodyDelayL35/1 -> BodySumL35/1, BodyDelayL36/1
  BodySumL35/1 -> h(35)/1
  h(35)/1 -> BodySumR35/1
  BodyDelayR35/1 -> BodySumL35/2, BodyDelayR34/1
  BodySumR35/1 -> BodySumR36/2
  BodyDelayL36/1 -> BodySumL36/1, BodyDelayL37/1
  BodySumL36/1 -> h(36)/1
  h(36)/1 -> BodySumR36/1
  BodyDelayR36/1 -> BodySumL36/2, BodyDelayR35/1
  BodySumR36/1 -> BodySumR37/2
  BodyDelayL37/1 -> BodySumL37/1, BodyDelayL38/1
  BodySumL37/1 -> h(37)/1
  h(37)/1 -> BodySumR37/1
  BodyDelayR37/1 -> BodySumL37/2, BodyDelayR36/1
  BodySumR37/1 -> BodySumR38/2
  BodyDelayL38/1 -> BodySumL38/1, BodyDelayL39/1
  BodySumL38/1 -> h(38)/1
  h(38)/1 -> BodySumR38/1
  BodyDelayR38/1 -> BodySumL38/2, BodyDelayR37/1
  BodySumR38/1 -> BodySumR39/2
  BodyDelayL39/1 -> BodySumL39/1, BodyDelayL40/1
  BodySumL39/1 -> h(39)/1
  h(39)/1 -> BodySumR39/1
  BodyDelayR39/1 -> BodySumL39/2, BodyDelayR38/1
  BodySumR39/1 -> BodySumR40/2
  BodyDelayL40/1 -> BodySumL40/1, BodyDelayL41/1
  BodySumL40/1 -> h(40)/1
  h(40)/1 -> BodySumR40/1
  BodyDelayR40/1 -> BodySumL40/2, BodyDelayR39/1
  BodySumR40/1 -> BodySumR41/2
  BodyDelayL41/1 -> BodySumL41/1, BodyDelayL42/1
  BodySumL41/1 -> h(41)/1
  h(41)/1 -> BodySumR41/1
  BodyDelayR41/1 -> BodySumL41/2, BodyDelayR40/1
  BodySumR41/1 -> BodySumR42/2
  BodyDelayL42/1 -> BodySumL42/1, BodyDelayL43/1
  BodySumL42/1 -> h(42)/1
  h(42)/1 -> BodySumR42/1
  BodyDelayR42/1 -> BodySumL42/2, BodyDelayR41/1
  BodySumR42/1 -> BodySumR43/2
  BodyDelayL43/1 -> BodySumL43/1, BodyDelayL44/1
  BodySumL43/1 -> h(43)/1
  h(43)/1 -> BodySumR43/1
  BodyDelayR43/1 -> BodySumL43/2, BodyDelayR42/1
  BodySumR43/1 -> BodySumR44/2
  BodyDelayL44/1 -> BodySumL44/1, BodyDelayL45/1
  BodySumL44/1 -> h(44)/1
  h(44)/1 -> BodySumR44/1
  BodyDelayR44/1 -> BodySumL44/2, BodyDelayR43/1
  BodySumR44/1 -> BodySumR45/2
  BodyDelayL45/1 -> BodySumL45/1, BodyDelayL46/1
  BodySumL45/1 -> h(45)/1
  h(45)/1 -> BodySumR45/1
  BodyDelayR45/1 -> BodySumL45/2, BodyDelayR44/1
  BodySumR45/1 -> BodySumR46/2
  BodyDelayL46/1 -> BodySumL46/1, BodyDelayL47/1
  BodySumL46/1 -> h(46)/1
  h(46)/1 -> BodySumR46/1
  BodyDelayR46/1 -> BodySumL46/2, BodyDelayR45/1
  BodySumR46/1 -> BodySumR47/2
  BodyDelayL47/1 -> BodySumL47/1, BodyDelayL48/1
  BodySumL47/1 -> h(47)/1
  h(47)/1 -> BodySumR47/1
  BodyDelayR47/1 -> BodySumL47/2, BodyDelayR46/1
  BodySumR47/1 -> BodySumR48/2
  BodyDelayL48/1 -> BodySumL48/1, BodyDelayL49/1
  BodySumL48/1 -> h(48)/1
  h(48)/1 -> BodySumR48/1
  BodyDelayR48/1 -> BodySumL48/2, BodyDelayR47/1
  BodySumR48/1 -> BodySumR49/2
  BodyDelayL49/1 -> BodySumL49/1, BodyDelayL50/1
  BodySumL49/1 -> h(49)/1
  h(49)/1 -> BodySumR49/1
  BodyDelayR49/1 -> BodySumL49/2, BodyDelayR48/1
  BodySumR49/1 -> BodySumR50/2
  BodyDelayL50/1 -> BodySumL50/1, BodyDelayL51/1
  BodySumL50/1 -> h(50)/1
  h(50)/1 -> BodySumR50/1
  BodyDelayR50/1 -> BodySumL50/2, BodyDelayR49/1
  BodySumR50/1 -> BodySumR51/2
  BodyDelayL51/1 -> BodySumL51/1, BodyDelayL52/1
  BodySumL51/1 -> h(51)/1
  h(51)/1 -> BodySumR51/1
  BodyDelayR51/1 -> BodySumL51/2, BodyDelayR50/1
  BodySumR51/1 -> BodySumR52/2
  BodyDelayL52/1 -> BodySumL52/1, BodyDelayL53/1
  BodySumL52/1 -> h(52)/1
  h(52)/1 -> BodySumR52/1
  BodyDelayR52/1 -> BodySumL52/2, BodyDelayR51/1
  BodySumR52/1 -> BodySumR53/2
  BodyDelayL53/1 -> BodySumL53/1, BodyDelayL54/1
  BodySumL53/1 -> h(53)/1
  h(53)/1 -> BodySumR53/1
  BodyDelayR53/1 -> BodySumL53/2, BodyDelayR52/1
  BodySumR53/1 -> BodySumR54/2
  BodyDelayL54/1 -> BodySumL54/1, BodyDelayL55/1
  BodySumL54/1 -> h(54)/1
  h(54)/1 -> BodySumR54/1
  BodyDelayR54/1 -> BodySumL54/2, BodyDelayR53/1
  BodySumR54/1 -> BodySumR55/2
  BodyDelayL55/1 -> BodySumL55/1, BodyDelayL56/1
  BodySumL55/1 -> h(55)/1
  h(55)/1 -> BodySumR55/1
  BodyDelayR55/1 -> BodySumL55/2, BodyDelayR54/1
  BodySumR55/1 -> BodySumR56/2
  BodyDelayL56/1 -> BodySumL56/1, BodyDelayL57/1
  BodySumL56/1 -> h(56)/1
  h(56)/1 -> BodySumR56/1
  BodyDelayR56/1 -> BodySumL56/2, BodyDelayR55/1
  BodySumR56/1 -> BodySumR57/2
  BodyDelayL57/1 -> BodySumL57/1, BodyDelayL58/1
  BodySumL57/1 -> h(57)/1
  h(57)/1 -> BodySumR57/1
  BodyDelayR57/1 -> BodySumL57/2, BodyDelayR56/1
  BodySumR57/1 -> BodySumR58/2
  BodyDelayL58/1 -> BodySumL58/1, BodyDelayL59/1
  BodySumL58/1 -> h(58)/1
  h(58)/1 -> BodySumR58/1
  BodyDelayR58/1 -> BodySumL58/2, BodyDelayR57/1
  BodySumR58/1 -> BodySumR59/2
  BodyDelayL59/1 -> BodySumL59/1, BodyDelayL60/1
  BodySumL59/1 -> h(59)/1
  h(59)/1 -> BodySumR59/1
  BodyDelayR59/1 -> BodySumL59/2, BodyDelayR58/1
  BodySumR59/1 -> BodySumR60/2
  BodyDelayL60/1 -> BodySumL60/1, BodyDelayL61/1
  BodySumL60/1 -> h(60)/1
  h(60)/1 -> BodySumR60/1
  BodyDelayR60/1 -> BodySumL60/2, BodyDelayR59/1
  BodySumR60/1 -> BodySumR61/2
  BodyDelayL61/1 -> BodySumL61/1, BodyDelayL62/1
  BodySumL61/1 -> h(61)/1
  h(61)/1 -> BodySumR61/1
  BodyDelayR61/1 -> BodySumL61/2, BodyDelayR60/1
  BodySumR61/1 -> BodySumR62/2
  BodyDelayL62/1 -> BodySumL62/1, BodyDelayL63/1
  BodySumL62/1 -> h(62)/1
  h(62)/1 -> BodySumR62/1
  BodyDelayR62/1 -> BodySumL62/2, BodyDelayR61/1
  BodySumR62/1 -> BodySumR63/2
  BodyDelayL63/1 -> BodySumL63/1, BodyDelayL64/1
  BodySumL63/1 -> h(63)/1
  h(63)/1 -> BodySumR63/1
  BodyDelayR63/1 -> BodySumL63/2, BodyDelayR62/1
  BodySumR63/1 -> BodySumR64/2
  BodyDelayL64/1 -> BodySumL64/1, BodyDelayL65/1
  BodySumL64/1 -> h(64)/1
  h(64)/1 -> BodySumR64/1
  BodyDelayR64/1 -> BodySumL64/2, BodyDelayR63/1
  BodySumR64/1 -> BodySumR65/2
  BodyDelayL65/1 -> BodySumL65/1, BodyDelayL66/1
  BodySumL65/1 -> h(65)/1
  h(65)/1 -> BodySumR65/1
  BodyDelayR65/1 -> BodySumL65/2, BodyDelayR64/1
  BodySumR65/1 -> BodySumR66/2
  BodyDelayL66/1 -> BodySumL66/1, BodyDelayL67/1
  BodySumL66/1 -> h(66)/1
  h(66)/1 -> BodySumR66/1
  BodyDelayR66/1 -> BodySumL66/2, BodyDelayR65/1
  BodySumR66/1 -> BodySumR67/2
  BodyDelayL67/1 -> BodySumL67/1, BodyDelayL68/1
  BodySumL67/1 -> h(67)/1
  h(67)/1 -> BodySumR67/1
  BodyDelayR67/1 -> BodySumL67/2, BodyDelayR66/1
  BodySumR67/1 -> BodySumR68/2
  BodyDelayL68/1 -> BodySumL68/1, BodyDelayL69/1
  BodySumL68/1 -> h(68)/1
  h(68)/1 -> BodySumR68/1
  BodyDelayR68/1 -> BodySumL68/2, BodyDelayR67/1
  BodySumR68/1 -> BodySumR69/2
  BodyDelayL69/1 -> BodySumL69/1, BodyDelayL70/1
  BodySumL69/1 -> h(69)/1
  h(69)/1 -> BodySumR69/1
  BodyDelayR69/1 -> BodySumL69/2, BodyDelayR68/1
  BodySumR69/1 -> BodySumR70/2
  BodyDelayL70/1 -> BodySumL70/1, BodyDelayL71/1
  BodySumL70/1 -> h(70)/1
  h(70)/1 -> BodySumR70/1
  BodyDelayR70/1 -> BodySumL70/2, BodyDelayR69/1
  BodySumR70/1 -> BodySumR71/2
  BodyDelayL71/1 -> BodySumL71/1, BodyDelayL72/1
  BodySumL71/1 -> h(71)/1
  h(71)/1 -> BodySumR71/1
  BodyDelayR71/1 -> BodySumL71/2, BodyDelayR70/1
  BodySumR71/1 -> BodySumR72/2
  BodyDelayL72/1 -> BodySumL72/1, BodyDelayL73/1
  BodySumL72/1 -> h(72)/1
  h(72)/1 -> BodySumR72/1
  BodyDelayR72/1 -> BodySumL72/2, BodyDelayR71/1
  BodySumR72/1 -> BodySumR73/2
  BodyDelayL73/1 -> BodySumL73/1, BodyDelayL74/1
  BodySumL73/1 -> h(73)/1
  h(73)/1 -> BodySumR73/1
  BodyDelayR73/1 -> BodySumL73/2, BodyDelayR72/1
  BodySumR73/1 -> BodySumR74/2
  BodyDelayL74/1 -> BodySumL74/1, BodyDelayL75/1
  BodySumL74/1 -> h(74)/1
  h(74)/1 -> BodySumR74/1
  BodyDelayR74/1 -> BodySumL74/2, BodyDelayR73/1
  BodySumR74/1 -> BodySumR75/2
  BodyDelayL75/1 -> BodySumL75/1, BodyDelayL76/1
  BodySumL75/1 -> h(75)/1
  h(75)/1 -> BodySumR75/1
  BodyDelayR75/1 -> BodySumL75/2, BodyDelayR74/1
  BodySumR75/1 -> BodySumR76/2
  BodyDelayL76/1 -> BodySumL76/1, BodyDelayL77/1
  BodySumL76/1 -> h(76)/1
  h(76)/1 -> BodySumR76/1
  BodyDelayR76/1 -> BodySumL76/2, BodyDelayR75/1
  BodySumR76/1 -> BodySumR77/2
  BodyDelayL77/1 -> BodySumL77/1, BodyDelayL78/1
  BodySumL77/1 -> h(77)/1
  h(77)/1 -> BodySumR77/1
  BodyDelayR77/1 -> BodySumL77/2, BodyDelayR76/1
  BodySumR77/1 -> BodySumR78/2
  BodyDelayL78/1 -> BodySumL78/1, BodyDelayL79/1
  BodySumL78/1 -> h(78)/1
  h(78)/1 -> BodySumR78/1
  BodyDelayR78/1 -> BodySumL78/2, BodyDelayR77/1
  BodySumR78/1 -> BodySumR79/2
  BodyDelayL79/1 -> BodySumL79/1, BodyDelayL80/1
  BodySumL79/1 -> h(79)/1
  h(79)/1 -> BodySumR79/1
  BodyDelayR79/1 -> BodySumL79/2, BodyDelayR78/1
  BodySumR79/1 -> BodySumR80/2
  BodyDelayL80/1 -> BodySumL80/1, BodyDelayL81/1
  BodySumL80/1 -> h(80)/1
  h(80)/1 -> BodySumR80/1
  BodyDelayR80/1 -> BodySumL80/2, BodyDelayR79/1
  BodySumR80/1 -> BodySumR81/2
  BodyDelayL81/1 -> BodySumL81/1, BodyDelayL82/1
  BodySumL81/1 -> h(81)/1
  h(81)/1 -> BodySumR81/1
  BodyDelayR81/1 -> BodySumL81/2, BodyDelayR80/1
  BodySumR81/1 -> BodySumR82/2
  BodyDelayL82/1 -> BodySumL82/1, BodyDelayL83/1
  BodySumL82/1 -> h(82)/1
  h(82)/1 -> BodySumR82/1
  BodyDelayR82/1 -> BodySumL82/2, BodyDelayR81/1
  BodySumR82/1 -> BodySumR83/2
  BodyDelayL83/1 -> BodySumL83/1, BodyDelayL84/1
  BodySumL83/1 -> h(83)/1
  h(83)/1 -> BodySumR83/1
  BodyDelayR83/1 -> BodySumL83/2, BodyDelayR82/1
  BodySumR83/1 -> BodySumR84/2
  BodyDelayL84/1 -> BodySumL84/1, BodyDelayL85/1
  BodySumL84/1 -> h(84)/1
  h(84)/1 -> BodySumR84/1
  BodyDelayR84/1 -> BodySumL84/2, BodyDelayR83/1
  BodySumR84/1 -> BodySumR85/2
  BodyDelayL85/1 -> BodySumL85/1, BodyDelayL86/1
  BodySumL85/1 -> h(85)/1
  h(85)/1 -> BodySumR85/1
  BodyDelayR85/1 -> BodySumL85/2, BodyDelayR84/1
  BodySumR85/1 -> BodySumR86/2
  BodyDelayL86/1 -> BodySumL86/1, BodyDelayL87/1
  BodySumL86/1 -> h(86)/1
  h(86)/1 -> BodySumR86/1
  BodyDelayR86/1 -> BodySumL86/2, BodyDelayR85/1
  BodySumR86/1 -> BodySumR87/2
  BodyDelayL87/1 -> BodySumL87/1, BodyDelayL88/1
  BodySumL87/1 -> h(87)/1
  h(87)/1 -> BodySumR87/1
  BodyDelayR87/1 -> BodySumL87/2, BodyDelayR86/1
  BodySumR87/1 -> BodySumR88/2
  BodyDelayL88/1 -> BodySumL88/1, BodyDelayL89/1
  BodySumL88/1 -> h(88)/1
  h(88)/1 -> BodySumR88/1
  BodyDelayR88/1 -> BodySumL88/2, BodyDelayR87/1
  BodySumR88/1 -> BodySumR89/2
  BodyDelayL89/1 -> BodySumL89/1, BodyDelayL90/1
  BodySumL89/1 -> h(89)/1
  h(89)/1 -> BodySumR89/1
  BodyDelayR89/1 -> BodySumL89/2, BodyDelayR88/1
  BodySumR89/1 -> BodySumR90/2
  BodyDelayL90/1 -> BodySumL90/1, BodyDelayL91/1
  BodySumL90/1 -> h(90)/1
  h(90)/1 -> BodySumR90/1
  BodyDelayR90/1 -> BodySumL90/2, BodyDelayR89/1
  BodySumR90/1 -> BodySumR91/2
  BodyDelayL91/1 -> BodySumL91/1, BodyDelayL92/1
  BodySumL91/1 -> h(91)/1
  h(91)/1 -> BodySumR91/1
  BodyDelayR91/1 -> BodySumL91/2, BodyDelayR90/1
  BodySumR91/1 -> BodySumR92/2
  BodyDelayL92/1 -> BodySumL92/1, BodyDelayL93/1
  BodySumL92/1 -> h(92)/1
  h(92)/1 -> BodySumR92/1
  BodyDelayR92/1 -> BodySumL92/2, BodyDelayR91/1
  BodySumR92/1 -> BodySumR93/2
  BodyDelayL93/1 -> BodySumL93/1, BodyDelayL94/1
  BodySumL93/1 -> h(93)/1
  h(93)/1 -> BodySumR93/1
  BodyDelayR93/1 -> BodySumL93/2, BodyDelayR92/1
  BodySumR93/1 -> BodySumR94/2
  BodyDelayL94/1 -> BodySumL94/1, BodyDelayL95/1
  BodySumL94/1 -> h(94)/1
  h(94)/1 -> BodySumR94/1
  BodyDelayR94/1 -> BodySumL94/2, BodyDelayR93/1
  BodySumR94/1 -> BodySumR95/2
  BodyDelayL95/1 -> BodySumL95/1, BodyDelayL96/1
  BodySumL95/1 -> h(95)/1
  h(95)/1 -> BodySumR95/1
  BodyDelayR95/1 -> BodySumL95/2, BodyDelayR94/1
  BodySumR95/1 -> BodySumR96/2
  BodyDelayL96/1 -> BodySumL96/1, BodyDelayL97/1
  BodySumL96/1 -> h(96)/1
  h(96)/1 -> BodySumR96/1
  BodyDelayR96/1 -> BodySumL96/2, BodyDelayR95/1
  BodySumR96/1 -> BodySumR97/2
  BodyDelayL97/1 -> BodySumL97/1, BodyDelayL98/1
  BodySumL97/1 -> h(97)/1
  h(97)/1 -> BodySumR97/1
  BodyDelayR97/1 -> BodySumL97/2, BodyDelayR96/1
  BodySumR97/1 -> BodySumR98/2
  BodyDelayL98/1 -> BodySumL98/1, BodyDelayL99/1
  BodySumL98/1 -> h(98)/1
  h(98)/1 -> BodySumR98/1
  BodyDelayR98/1 -> BodySumL98/2, BodyDelayR97/1
  BodySumR98/1 -> BodySumR99/2
  BodyDelayL99/1 -> BodySumL99/1, BodyDelayL100/1
  BodySumL99/1 -> h(99)/1
  h(99)/1 -> BodySumR99/1
  BodyDelayR99/1 -> BodySumL99/2, BodyDelayR98/1
  BodySumR99/1 -> BodySumR100/2
  BodyDelayL100/1 -> BodySumL100/1, BodyDelayL101/1
  BodySumL100/1 -> h(100)/1
  h(100)/1 -> BodySumR100/1
  BodyDelayR100/1 -> BodySumL100/2, BodyDelayR99/1
  BodySumR100/1 -> BodySumR101/2
  BodyDelayL101/1 -> BodySumL101/1, BodyDelayL102/1
  BodySumL101/1 -> h(101)/1
  h(101)/1 -> BodySumR101/1
  BodyDelayR101/1 -> BodySumL101/2, BodyDelayR100/1
  BodySumR101/1 -> BodySumR102/2
  BodyDelayL102/1 -> BodySumL102/1, BodyDelayL103/1
  BodySumL102/1 -> h(102)/1
  h(102)/1 -> BodySumR102/1
  BodyDelayR102/1 -> BodySumL102/2, BodyDelayR101/1
  BodySumR102/1 -> BodySumR103/2
  BodyDelayL103/1 -> BodySumL103/1, BodyDelayL104/1
  BodySumL103/1 -> h(103)/1
  h(103)/1 -> BodySumR103/1
  BodyDelayR103/1 -> BodySumL103/2, BodyDelayR102/1
  BodySumR103/1 -> BodySumR104/2
  BodyDelayL104/1 -> BodySumL104/1, BodyDelayL105/1
  BodySumL104/1 -> h(104)/1
  h(104)/1 -> BodySumR104/1
  BodyDelayR104/1 -> BodySumL104/2, BodyDelayR103/1
  BodySumR104/1 -> BodySumR105/2
  BodyDelayL105/1 -> BodySumL105/1, BodyDelayL106/1
  BodySumL105/1 -> h(105)/1
  h(105)/1 -> BodySumR105/1
  BodyDelayR105/1 -> BodySumL105/2, BodyDelayR104/1
  BodySumR105/1 -> BodySumR106/2
  BodyDelayL106/1 -> BodySumL106/1, BodyDelayL107/1
  BodySumL106/1 -> h(106)/1
  h(106)/1 -> BodySumR106/1
  BodyDelayR106/1 -> BodySumL106/2, BodyDelayR105/1
  BodySumR106/1 -> BodySumR107/2
  BodyDelayL107/1 -> BodySumL107/1, BodyDelayL108/1
  BodySumL107/1 -> h(107)/1
  h(107)/1 -> BodySumR107/1
  BodyDelayR107/1 -> BodySumL107/2, BodyDelayR106/1
  BodySumR107/1 -> BodySumR108/2
  BodyDelayL108/1 -> BodySumL108/1, BodyDelayL109/1
  BodySumL108/1 -> h(108)/1
  h(108)/1 -> BodySumR108/1
  BodyDelayR108/1 -> BodySumL108/2, BodyDelayR107/1
  BodySumR108/1 -> BodySumR109/2
  BodyDelayL109/1 -> BodySumL109/1, BodyDelayL110/1
  BodySumL109/1 -> h(109)/1
  h(109)/1 -> BodySumR109/1
  BodyDelayR109/1 -> BodySumL109/2, BodyDelayR108/1
  BodySumR109/1 -> BodySumR110/2
  BodyDelayL110/1 -> BodySumL110/1, BodyDelayL111/1
  BodySumL110/1 -> h(110)/1
  h(110)/1 -> BodySumR110/1
  BodyDelayR110/1 -> BodySumL110/2, BodyDelayR109/1
  BodySumR110/1 -> BodySumR111/2
  BodyDelayL111/1 -> BodySumL111/1, BodyDelayL112/1
  BodySumL111/1 -> h(111)/1
  h(111)/1 -> BodySumR111/1
  BodyDelayR111/1 -> BodySumL111/2, BodyDelayR110/1
  BodySumR111/1 -> BodySumR112/2
  BodyDelayL112/1 -> BodySumL112/1, BodyDelayL113/1
  BodySumL112/1 -> h(112)/1
  h(112)/1 -> BodySumR112/1
  BodyDelayR112/1 -> BodySumL112/2, BodyDelayR111/1
  BodySumR112/1 -> BodySumR113/2
  BodyDelayL113/1 -> BodySumL113/1, BodyDelayL114/1
  BodySumL113/1 -> h(113)/1
  h(113)/1 -> BodySumR113/1
  BodyDelayR113/1 -> BodySumL113/2, BodyDelayR112/1
  BodySumR113/1 -> BodySumR114/2
  BodyDelayL114/1 -> BodySumL114/1, BodyDelayL115/1
  BodySumL114/1 -> h(114)/1
  h(114)/1 -> BodySumR114/1
  BodyDelayR114/1 -> BodySumL114/2, BodyDelayR113/1
  BodySumR114/1 -> BodySumR115/2
  BodyDelayL115/1 -> BodySumL115/1, BodyDelayL116/1
  BodySumL115/1 -> h(115)/1
  h(115)/1 -> BodySumR115/1
  BodyDelayR115/1 -> BodySumL115/2, BodyDelayR114/1
  BodySumR115/1 -> BodySumR116/2
  BodyDelayL116/1 -> BodySumL116/1, BodyDelayL117/1
  BodySumL116/1 -> h(116)/1
  h(116)/1 -> BodySumR116/1
  BodyDelayR116/1 -> BodySumL116/2, BodyDelayR115/1
  BodySumR116/1 -> BodySumR117/2
  BodyDelayL117/1 -> BodySumL117/1, BodyDelayL118/1
  BodySumL117/1 -> h(117)/1
  h(117)/1 -> BodySumR117/1
  BodyDelayR117/1 -> BodySumL117/2, BodyDelayR116/1
  BodySumR117/1 -> BodySumR118/2
  BodyDelayL118/1 -> BodySumL118/1, BodyDelayL119/1
  BodySumL118/1 -> h(118)/1
  h(118)/1 -> BodySumR118/1
  BodyDelayR118/1 -> BodySumL118/2, BodyDelayR117/1
  BodySumR118/1 -> BodySumR119/2
  BodyDelayL119/1 -> BodySumL119/1, BodyDelayL120/1
  BodySumL119/1 -> h(119)/1
  h(119)/1 -> BodySumR119/1
  BodyDelayR119/1 -> BodySumL119/2, BodyDelayR118/1
  BodySumR119/1 -> BodySumR120/2
  BodyDelayL120/1 -> BodySumL120/1, BodyDelayL121/1
  BodySumL120/1 -> h(120)/1
  h(120)/1 -> BodySumR120/1
  BodyDelayR120/1 -> BodySumL120/2, BodyDelayR119/1
  BodySumR120/1 -> BodySumR121/2
  BodyDelayL121/1 -> BodySumL121/1, BodyDelayL122/1
  BodySumL121/1 -> h(121)/1
  h(121)/1 -> BodySumR121/1
  BodyDelayR121/1 -> BodySumL121/2, BodyDelayR120/1
  BodySumR121/1 -> BodySumR122/2
  BodyDelayL122/1 -> BodySumL122/1, BodyDelayL123/1
  BodySumL122/1 -> h(122)/1
  h(122)/1 -> BodySumR122/1
  BodyDelayR122/1 -> BodySumL122/2, BodyDelayR121/1
  BodySumR122/1 -> BodySumR123/2
  BodyDelayL123/1 -> BodySumL123/1, BodyDelayL124/1
  BodySumL123/1 -> h(123)/1
  h(123)/1 -> BodySumR123/1
  BodyDelayR123/1 -> BodySumL123/2, BodyDelayR122/1
  BodySumR123/1 -> BodySumR124/2
  BodyDelayL124/1 -> BodySumL124/1, BodyDelayL125/1
  BodySumL124/1 -> h(124)/1
  h(124)/1 -> BodySumR124/1
  BodyDelayR124/1 -> BodySumL124/2, BodyDelayR123/1
  BodySumR124/1 -> BodySumR125/2
  BodyDelayL125/1 -> BodySumL125/1, BodyDelayL126/1
  BodySumL125/1 -> h(125)/1
  h(125)/1 -> BodySumR125/1
  BodyDelayR125/1 -> BodySumL125/2, BodyDelayR124/1
  BodySumR125/1 -> BodySumR126/2
  BodyDelayL126/1 -> BodySumL126/1, BodyDelayL127/1
  BodySumL126/1 -> h(126)/1
  h(126)/1 -> BodySumR126/1
  BodyDelayR126/1 -> BodySumL126/2, BodyDelayR125/1
  BodySumR126/1 -> BodySumR127/2
  BodyDelayL127/1 -> BodySumL127/1, BodyDelayL128/1
  BodySumL127/1 -> h(127)/1
  h(127)/1 -> BodySumR127/1
  BodyDelayR127/1 -> BodySumL127/2, BodyDelayR126/1
  BodySumR127/1 -> BodySumR128/2
  BodyDelayL128/1 -> BodySumL128/1, BodyDelayL129/1
  BodySumL128/1 -> h(128)/1
  h(128)/1 -> BodySumR128/1
  BodyDelayR128/1 -> BodySumL128/2, BodyDelayR127/1
  BodySumR128/1 -> BodySumR129/2
  BodyDelayL129/1 -> BodySumL129/1, BodyDelayL130/1
  BodySumL129/1 -> h(129)/1
  h(129)/1 -> BodySumR129/1
  BodyDelayR129/1 -> BodySumL129/2, BodyDelayR128/1
  BodySumR129/1 -> BodySumR130/2
  BodyDelayL130/1 -> BodySumL130/1, BodyDelayL131/1
  BodySumL130/1 -> h(130)/1
  h(130)/1 -> BodySumR130/1
  BodyDelayR130/1 -> BodySumL130/2, BodyDelayR129/1
  BodySumR130/1 -> BodySumR131/2
  BodyDelayL131/1 -> BodySumL131/1, BodyDelayL132/1
  BodySumL131/1 -> h(131)/1
  h(131)/1 -> BodySumR131/1
  BodyDelayR131/1 -> BodySumL131/2, BodyDelayR130/1
  BodySumR131/1 -> BodySumR132/2
  BodyDelayL132/1 -> BodySumL132/1, BodyDelayL133/1
  BodySumL132/1 -> h(132)/1
  h(132)/1 -> BodySumR132/1
  BodyDelayR132/1 -> BodySumL132/2, BodyDelayR131/1
  BodySumR132/1 -> BodySumR133/2
  BodyDelayL133/1 -> BodySumL133/1, BodyDelayL134/1
  BodySumL133/1 -> h(133)/1
  h(133)/1 -> BodySumR133/1
  BodyDelayR133/1 -> BodySumL133/2, BodyDelayR132/1
  BodySumR133/1 -> BodySumR134/2
  BodyDelayL134/1 -> BodySumL134/1, BodyDelayL135/1
  BodySumL134/1 -> h(134)/1
  h(134)/1 -> BodySumR134/1
  BodyDelayR134/1 -> BodySumL134/2, BodyDelayR133/1
  BodySumR134/1 -> BodySumR135/2
  BodyDelayL135/1 -> BodySumL135/1, BodyDelayL136/1
  BodySumL135/1 -> h(135)/1
  h(135)/1 -> BodySumR135/1
  BodyDelayR135/1 -> BodySumL135/2, BodyDelayR134/1
  BodySumR135/1 -> BodySumR136/2
  BodyDelayL136/1 -> BodySumL136/1, BodyDelayL137/1
  BodySumL136/1 -> h(136)/1
  h(136)/1 -> BodySumR136/1
  BodyDelayR136/1 -> BodySumL136/2, BodyDelayR135/1
  BodySumR136/1 -> BodySumR137/2
  BodyDelayL137/1 -> BodySumL137/1, BodyDelayL138/1
  BodySumL137/1 -> h(137)/1
  h(137)/1 -> BodySumR137/1
  BodyDelayR137/1 -> BodySumL137/2, BodyDelayR136/1
  BodySumR137/1 -> BodySumR138/2
  BodyDelayL138/1 -> BodySumL138/1, BodyDelayL139/1
  BodySumL138/1 -> h(138)/1
  h(138)/1 -> BodySumR138/1
  BodyDelayR138/1 -> BodySumL138/2, BodyDelayR137/1
  BodySumR138/1 -> BodySumR139/2
  BodyDelayL139/1 -> BodySumL139/1, BodyDelayL140/1
  BodySumL139/1 -> h(139)/1
  h(139)/1 -> BodySumR139/1
  BodyDelayR139/1 -> BodySumL139/2, BodyDelayR138/1
  BodySumR139/1 -> BodySumR140/2
  BodyDelayL140/1 -> BodySumL140/1, BodyDelayL141/1
  BodySumL140/1 -> h(140)/1
  h(140)/1 -> BodySumR140/1
  BodyDelayR140/1 -> BodySumL140/2, BodyDelayR139/1
  BodySumR140/1 -> BodySumR141/2
  BodyDelayL141/1 -> BodySumL141/1, BodyDelayL142/1
  BodySumL141/1 -> h(141)/1
  h(141)/1 -> BodySumR141/1
  BodyDelayR141/1 -> BodySumL141/2, BodyDelayR140/1
  BodySumR141/1 -> BodySumR142/2
  BodyDelayL142/1 -> BodySumL142/1, BodyDelayL143/1
  BodySumL142/1 -> h(142)/1
  h(142)/1 -> BodySumR142/1
  BodyDelayR142/1 -> BodySumL142/2, BodyDelayR141/1
  BodySumR142/1 -> BodySumR143/2
  BodyDelayL143/1 -> BodySumL143/1, BodyDelayL144/1
  BodySumL143/1 -> h(143)/1
  h(143)/1 -> BodySumR143/1
  BodyDelayR143/1 -> BodySumL143/2, BodyDelayR142/1
  BodySumR143/1 -> BodySumR144/2
  BodyDelayL144/1 -> BodySumL144/1, BodyDelayL145/1
  BodySumL144/1 -> h(144)/1
  h(144)/1 -> BodySumR144/1
  BodyDelayR144/1 -> BodySumL144/2, BodyDelayR143/1
  BodySumR144/1 -> BodySumR145/2
  BodyDelayL145/1 -> BodySumL145/1, BodyDelayL146/1
  BodySumL145/1 -> h(145)/1
  h(145)/1 -> BodySumR145/1
  BodyDelayR145/1 -> BodySumL145/2, BodyDelayR144/1
  BodySumR145/1 -> BodySumR146/2
  BodyDelayL146/1 -> BodySumL146/1, BodyDelayL147/1
  BodySumL146/1 -> h(146)/1
  h(146)/1 -> BodySumR146/1
  BodyDelayR146/1 -> BodySumL146/2, BodyDelayR145/1
  BodySumR146/1 -> BodySumR147/2
  BodyDelayL147/1 -> BodySumL147/1, BodyDelayL148/1
  BodySumL147/1 -> h(147)/1
  h(147)/1 -> BodySumR147/1
  BodyDelayR147/1 -> BodySumL147/2, BodyDelayR146/1
  BodySumR147/1 -> BodySumR148/2
  BodyDelayL148/1 -> BodySumL148/1, BodyDelayL149/1
  BodySumL148/1 -> h(148)/1
  h(148)/1 -> BodySumR148/1
  BodyDelayR148/1 -> BodySumL148/2, BodyDelayR147/1
  BodySumR148/1 -> BodySumR149/2
  BodyDelayL149/1 -> BodySumL149/1, BodyDelayL150/1
  BodySumL149/1 -> h(149)/1
  h(149)/1 -> BodySumR149/1
  BodyDelayR149/1 -> BodySumL149/2, BodyDelayR148/1
  BodySumR149/1 -> BodySumR150/2
  BodyDelayL150/1 -> BodySumL150/1, BodyDelayL151/1
  BodySumL150/1 -> h(150)/1
  h(150)/1 -> BodySumR150/1
  BodyDelayR150/1 -> BodySumL150/2, BodyDelayR149/1
  BodySumR150/1 -> BodySumR151/2
  BodyDelayL151/1 -> BodySumL151/1, BodyDelayL152/1
  BodySumL151/1 -> h(151)/1
  h(151)/1 -> BodySumR151/1
  BodyDelayR151/1 -> BodySumL151/2, BodyDelayR150/1
  BodySumR151/1 -> BodySumR152/2
  BodyDelayL152/1 -> BodySumL152/1, BodyDelayL153/1
  BodySumL152/1 -> h(152)/1
  h(152)/1 -> BodySumR152/1
  BodyDelayR152/1 -> BodySumL152/2, BodyDelayR151/1
  BodySumR152/1 -> BodySumR153/2
  BodyDelayL153/1 -> BodySumL153/1, BodyDelayL154/1
  BodySumL153/1 -> h(153)/1
  h(153)/1 -> BodySumR153/1
  BodyDelayR153/1 -> BodySumL153/2, BodyDelayR152/1
  BodySumR153/1 -> BodySumR154/2
  BodyDelayL154/1 -> BodySumL154/1, BodyDelayL155/1
  BodySumL154/1 -> h(154)/1
  h(154)/1 -> BodySumR154/1
  BodyDelayR154/1 -> BodySumL154/2, BodyDelayR153/1
  BodySumR154/1 -> BodySumR155/2
  BodyDelayL155/1 -> BodySumL155/1, BodyDelayL156/1
  BodySumL155/1 -> h(155)/1
  h(155)/1 -> BodySumR155/1
  BodyDelayR155/1 -> BodySumL155/2, BodyDelayR154/1
  BodySumR155/1 -> BodySumR156/2
  BodyDelayL156/1 -> BodySumL156/1, BodyDelayL157/1
  BodySumL156/1 -> h(156)/1
  h(156)/1 -> BodySumR156/1
  BodyDelayR156/1 -> BodySumL156/2, BodyDelayR155/1
  BodySumR156/1 -> BodySumR157/2
  BodyDelayL157/1 -> BodySumL157/1, BodyDelayL158/1
  BodySumL157/1 -> h(157)/1
  h(157)/1 -> BodySumR157/1
  BodyDelayR157/1 -> BodySumL157/2, BodyDelayR156/1
  BodySumR157/1 -> BodySumR158/2
  BodyDelayL158/1 -> BodySumL158/1, BodyDelayL159/1
  BodySumL158/1 -> h(158)/1
  h(158)/1 -> BodySumR158/1
  BodyDelayR158/1 -> BodySumL158/2, BodyDelayR157/1
  BodySumR158/1 -> BodySumR159/2
  BodyDelayL159/1 -> BodySumL159/1, BodyDelayL160/1
  BodySumL159/1 -> h(159)/1
  h(159)/1 -> BodySumR159/1
  BodyDelayR159/1 -> BodySumL159/2, BodyDelayR158/1
  BodySumR159/1 -> BodySumR160/2
  BodyDelayL160/1 -> BodySumL160/1, BodyDelayL161/1
  BodySumL160/1 -> h(160)/1
  h(160)/1 -> BodySumR160/1
  BodyDelayR160/1 -> BodySumL160/2, BodyDelayR159/1
  BodySumR160/1 -> BodySumR161/2
  BodyDelayL161/1 -> BodySumL161/1, BodyDelayL162/1
  BodySumL161/1 -> h(161)/1
  h(161)/1 -> BodySumR161/1
  BodyDelayR161/1 -> BodySumL161/2, BodyDelayR160/1
  BodySumR161/1 -> BodySumR162/2
  BodyDelayL162/1 -> BodySumL162/1, BodyDelayL163/1
  BodySumL162/1 -> h(162)/1
  h(162)/1 -> BodySumR162/1
  BodyDelayR162/1 -> BodySumL162/2, BodyDelayR161/1
  BodySumR162/1 -> BodySumR163/2
  BodyDelayL163/1 -> BodySumL163/1, BodyDelayL164/1
  BodySumL163/1 -> h(163)/1
  h(163)/1 -> BodySumR163/1
  BodyDelayR163/1 -> BodySumL163/2, BodyDelayR162/1
  BodySumR163/1 -> BodySumR164/2
  BodyDelayL164/1 -> BodySumL164/1, BodyDelayL165/1
  BodySumL164/1 -> h(164)/1
  h(164)/1 -> BodySumR164/1
  BodyDelayR164/1 -> BodySumL164/2, BodyDelayR163/1
  BodySumR164/1 -> BodySumR165/2
  BodyDelayL165/1 -> BodySumL165/1, BodyDelayL166/1
  BodySumL165/1 -> h(165)/1
  h(165)/1 -> BodySumR165/1
  BodyDelayR165/1 -> BodySumL165/2, BodyDelayR164/1
  BodySumR165/1 -> BodySumR166/2
  BodyDelayL166/1 -> BodySumL166/1, BodyDelayL167/1
  BodySumL166/1 -> h(166)/1
  h(166)/1 -> BodySumR166/1
  BodyDelayR166/1 -> BodySumL166/2, BodyDelayR165/1
  BodySumR166/1 -> BodySumR167/2
  BodyDelayL167/1 -> BodySumL167/1, BodyDelayL168/1
  BodySumL167/1 -> h(167)/1
  h(167)/1 -> BodySumR167/1
  BodyDelayR167/1 -> BodySumL167/2, BodyDelayR166/1
  BodySumR167/1 -> BodySumR168/2
  BodyDelayL168/1 -> BodySumL168/1, BodyDelayL169/1
  BodySumL168/1 -> h(168)/1
  h(168)/1 -> BodySumR168/1
  BodyDelayR168/1 -> BodySumL168/2, BodyDelayR167/1
  BodySumR168/1 -> BodySumR169/2
  BodyDelayL169/1 -> BodySumL169/1, BodyDelayL170/1
  BodySumL169/1 -> h(169)/1
  h(169)/1 -> BodySumR169/1
  BodyDelayR169/1 -> BodySumL169/2, BodyDelayR168/1
  BodySumR169/1 -> BodySumR170/2
  BodyDelayL170/1 -> BodySumL170/1, BodyDelayL171/1
  BodySumL170/1 -> h(170)/1
  h(170)/1 -> BodySumR170/1
  BodyDelayR170/1 -> BodySumL170/2, BodyDelayR169/1
  BodySumR170/1 -> BodySumR171/2
  BodyDelayL171/1 -> BodySumL171/1, FootDelayL172/1
  BodySumL171/1 -> h(171)/1
  h(171)/1 -> BodySumR171/1
  BodyDelayR171/1 -> BodySumL171/2, BodyDelayR170/1
  BodySumR171/1 -> FootSumR172/2
  FootDelayL172/1 -> h(172)/1, BodyDelayR171/1
  h(172)/1 -> FootSumR172/1
  FootSumR172/1 -> ConvertOut/1
  ConvertOut/1 -> Output/1
